simulink model "modelMain"  (R2021a)
settings: Solver=VariableStepAuto  StartTime=0.0  StopTime=10.0  RelTol=1e-3
values from neighbouring files (symbols this model uses):
  gamma = [1, 1, 1]    [runSimulink.m]
undefined symbols (not defined in the file or in its folder): B, d, epsilon, O, R, u0, x0
settings Model: Creator=sylva  LastModifiedBy=antonioterpin
settings SolverCC: AlgebraicLoopSolver=TrustRegion
settings DebuggingCC: SFMachineParentedDataDiag=warning

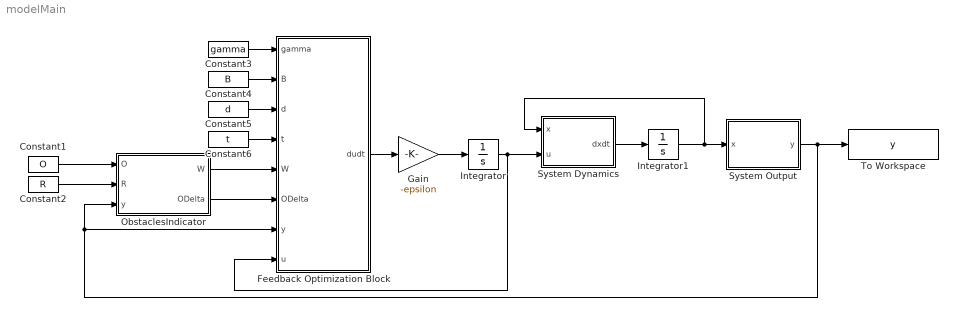
== system modelMain ==
  Constant1 : Constant  Value=O
  Constant2 : Constant  Value=R
  Constant3 : Constant  Value=gamma
  Constant4 : Constant  Value=B
  Constant5 : Constant  Value=d
  Constant6 : Constant  Value=t
  Feedback Optimization Block : MATLAB Function  TreatAsAtomicUnit=on
  Gain : Gain  Gain=-epsilon
  Integrator : Integrator  InitialCondition=u0
  Integrator1 : Integrator  InitialCondition=x0
  ObstaclesIndicator : MATLAB Function  TreatAsAtomicUnit=on
  System Dynamics : MATLAB Function  TreatAsAtomicUnit=on
  System Output : MATLAB Function  TreatAsAtomicUnit=on
  To Workspace : ToWorkspace  VariableName=y  SaveFormat=Timeseries  SampleTime=-1
  wires:
  Feedback Optimization Block/1(dudt) -> Gain/1
  Gain/1 -> Integrator/1
  Integrator/1 -> Feedback Optimization Block/8(u), System Dynamics/2(u)
  System Dynamics/1(dxdt) -> Integrator1/1
  Integrator1/1 -> System Dynamics/1(x), System Output/1(x)
  System Output/1(y) -> Feedback Optimization Block/7(y), ObstaclesIndicator/3(y), To Workspace/1
  Constant3/1 -> Feedback Optimization Block/1(gamma)
  Constant2/1 -> ObstaclesIndicator/2(R)
  Constant1/1 -> ObstaclesIndicator/1(O)
  ObstaclesIndicator/2(ODelta) -> Feedback Optimization Block/6(ODelta)
  ObstaclesIndicator/1(W) -> Feedback Optimization Block/5(W)
  Constant4/1 -> Feedback Optimization Block/2(B)
  Constant5/1 -> Feedback Optimization Block/3(d)
  Constant6/1 -> Feedback Optimization Block/4(t)

== matlab function modelMain/Feedback Optimization Block ==
  data: gamma input; B input; d input; t input; W input; ODelta input; y input; u input; dudt output
function dudt = ctrl(gamma, B, d, t, W, ODelta, y, u)
%CTRL Implements the feedback optimization controller
%   INPUT:
%       y       -- 2Nx1 positions of the agents [.., yix, yiy, ..].'
%       u       -- 2Nx1 Inputs
%       gamma   -- Gains of the cost function
%       B       -- Incidence matrix, the direction is specified implicitly
%                  through the cost function
%       d       -- 2size(B,2)x1 formation specification [.., dijx, dijy, ..].', 
%                  where the order of the edges is coherent with B
%       t       -- 2x1 target position
%       W       -- Number of obstacles detected by each agent
%       ODelta  -- Obstacle positions * Indicator matrix
%   OUTPUT:
%       dudt -- 2Nx1 gradient flow [.., duixdt, duiydt, ..].'

dudt = ...
    -gamma(1) * (kron(B*B.',eye(2)) * y - kron(B,eye(2)) * d) ...
    -gamma(2) * (y - repmat(t, numel(y) / 2, 1)) ...
    -gamma(3) * (W * y - ODelta);
end

== matlab function modelMain/System Dynamics ==
  data: x input; u input; dxdt output
function dxdt = dyn(x, u)
%DYN Implements the plant dynamics
%   INPUT:
%       x -- 3Nx1 agents state
%       u -- 2Nx1 agents input

N = numel(x) / 3;
k = [.1, -.1];
velSat = [-.1, .1];

% llc
ubar = zeros(2,N);
states = reshape(x,3,N);
delta = reshape(u,2,N) - states(1:2,:);
if any(delta ~= 0)
    theta = states(3,:) - atan2(delta(2,:), delta(1,:));
    ubar(1,:) = k(1) * vecnorm(delta,2,1) .* cos(theta);
    ubar(2,:) = -k(2) * theta;
end

% input saturation
vel = max(velSat(1), min(velSat(2), ubar(1,:)));
angVel = ubar(2,:);

% dxdt
dir = [cos(states(3,:)); sin(states(3,:))];
dxdt = reshape([repmat(vel,2,1) .* dir; angVel], [], 1);
end

== matlab function modelMain/System Output ==
  data: x input; y output
function y = fcn(x)
state = reshape(x,3,[]);
y = reshape(state(1:2,:), [], 1);
end

== matlab function modelMain/ObstaclesIndicator ==
  data: W output; O input; R input; y input; ODelta output
function [W,ODelta] = obst(O,R,y)
%OBST Implements the obstacles indicator matrix
%   INPUT:
%       y       -- 2Nx1 agents positions
%       O       -- 2xO obstacle positions
%       R       -- sensing radius
%   OUTPUT:
%       ODelta   -- 2NOx1 (obstacle indicator matrix)*obstacles 
%       W       -- Nx1 number of obstacles for each agent
Delta = kron(vecnorm(reshape(repmat(y, size(O,2) - repmat(O, numel(y) / 2, 1), 2, []), 2, 1) < R, [1,1]).';
ODelta = Delta.'*kron(eye(numel(y)/2),O.');
W = sum(reshape(Delta, 2, []), 2);
end
